simulink model "generate_joint_position_motion"  (R2025a)
settings: Solver=FixedStepDiscrete  StartTime=0.0  StopTime=inf  FixedStep=0.01  RelTol=1e-3
PreLoadFcn:
  | frs = FrankaRobotSettings;
libraries: franka_simulink x1
settings Model: SimulationMode=external  ExtModeTrigDuration=10000  Creator=vasi_ko  LastModifiedBy=kvasios
settings SolverCC: ConcurrentTasks=on  AlgebraicLoopSolver=TrustRegion  AutoInsertRateTranBlk=on
settings DataIOCC: LimitDataPoints=on  SaveFormat=Array  ReturnWorkspaceOutputs=off
settings OptimizationCC: EnhancedBackFolding=on  PassReuseOutputArgsAs=Individual arguments  ZeroExternalMemoryAtStartup=off  ZeroInternalMemoryAtStartup=off  MaxStackSize=200000  OptimizeBlockOrder=speed  DifferentSizesBufferReuse=on  OptimizationCustomize=off  EfficientTunableParamExpr=on
settings DebuggingCC: SolverPrmCheckMsg=warning  ParameterTunabilityLossMsg=error  UnconnectedInputMsg=warning  UnconnectedOutputMsg=warning  UnconnectedLineMsg=warning  SFUnexpectedBacktrackingDiag=warning  SFNoUnconditionalDefaultTransitionDiag=warning  SFExecutionAtInitializationDiag=none  ArithmeticOperatorsInVariantConditions=warning
settings HardwareCC: ProdBitPerLong=64.0  ProdLargestAtomicInteger=LongLong  ProdLargestAtomicFloat=Double  ProdLongLongMode=on  ProdHWDeviceType=ARM Compatible->ARM Cortex-A (64-bit)
settings ModelReferenceCC: EnableRefExpFcnMdlSchedulingChecks=on  PropagateSignalLabelsOutOfModel=off
settings SFSimCC: SimUseLocalCustomCode=off  MATLABDynamicMemAlloc=off  CustomCodeUndefinedFunction=UseInterfaceOnly  SimTargetLang=C++  SimDLTargetLibrary=mkl-dnn
settings RTWCC: SystemTargetFile=ert.tlc  HardwareBoard=NVIDIA Jetson  TLCOptions="-aInlineSetEventsForThisBaseRateFcn=TLC_FALSE -aSuppressMultiTaskScheduler=TLC_FALSE  -aRateBasedStepFcn=0"  TemplateMakefile=ert_default_tmf  RTWVerbose=off  RTWUseLocalCustomCode=off  BuildConfiguration=Faster Runs  TargetLang=C++  GPUComputeCapability=3.5  DLArmComputeVersion=19.05  Description=Embedded Coder
settings CodeAppCC: ForceParamTrailComments=on  IgnoreCustomStorageClasses=off  OperatorAnnotations=on  SimulinkDataObjDesc=on  SFDataObjDesc=on  InsertBlockDesc=on
settings ERTTargetCC: ExtModeTransport=0.0  ExtModeMexFile=ext_comm  ExtModeIntrfLevel=Level1  InlinedParameterPlacement=Hierarchical  RootIOFormat=Structure reference  TargetLangStandard=C++14 (ISO)
settings ConfigComp: CovMetricSettings=dw  CovSaveCumulativeToWorkspaceVar=on  CovSaveSingleToWorkspaceVar=on  CovExternalEMLEnable=off  CovSFcnEnable=off

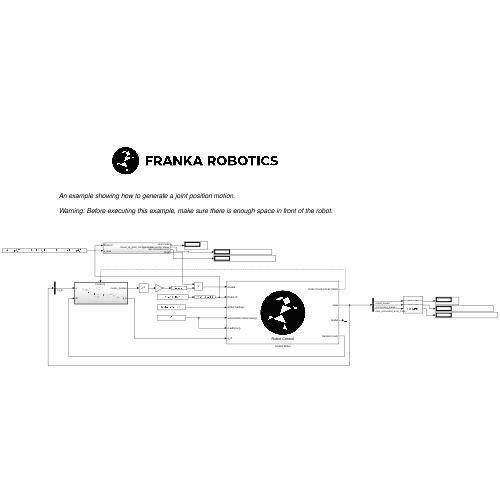
[thumbnail: Simulink's stored preview of the top-level diagram]
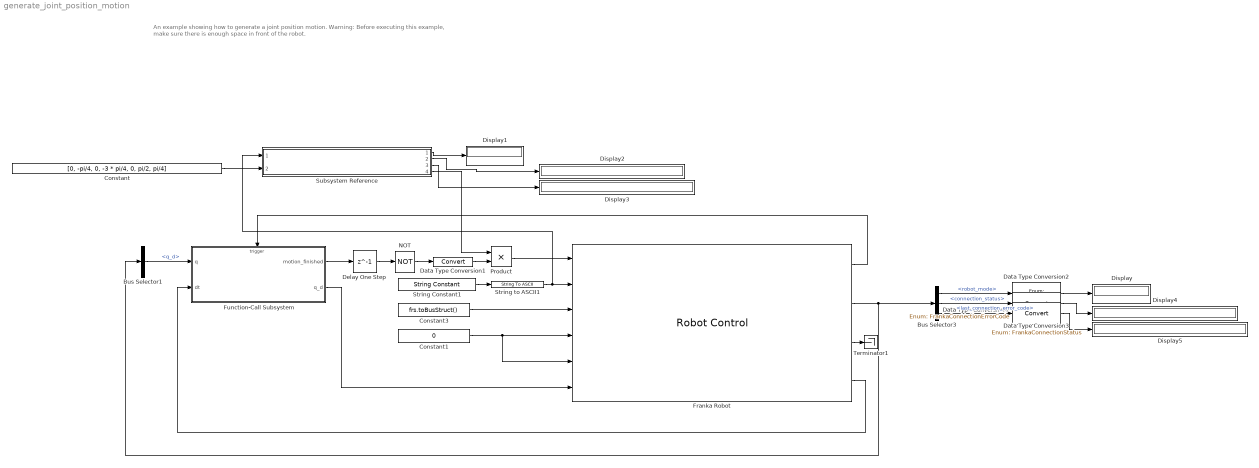
== system generate_joint_position_motion ==
  note: An example showing how to generate a joint position motion.
      |
      | Warning: Before executing this example, make sure there is enough space in front of the robot.
  Bus Selector1 : BusSelector  OutputSignals=q_d
  Bus Selector3 : BusSelector  OutputSignals=robot_mode,connection_status,last_connection_error_code
  Constant : Constant  Value=[0, -pi/4, 0, -3 * pi/4, 0, pi/2, pi/4]
  Constant1 : Constant  Value=0  OutDataTypeStr=Inherit: Inherit via back propagation
  Constant3 : Constant  Value=frs.toBusStruct()  OutDataTypeStr=Bus: FrankaRobotSettingsBus
  Data Type Conversion1 : DataTypeConversion  SaturateOnIntegerOverflow=off  RndMeth=Floor
  Data Type Conversion2 : DataTypeConversion  OutDataTypeStr=Enum: FrankaRobotModes  SaturateOnIntegerOverflow=off  RndMeth=Floor
  Data Type Conversion3 : DataTypeConversion  OutDataTypeStr=Enum: FrankaConnectionStatus  SaturateOnIntegerOverflow=off  RndMeth=Floor
  Data Type Conversion4 : DataTypeConversion  OutDataTypeStr=Enum: FrankaConnectionErrorCode  SaturateOnIntegerOverflow=off  RndMeth=Floor
  Delay One Step : Delay  DelayLength=1
  Display{,1..5} (6 alike) : Display
  Franka Robot : franka_simulink/Robot Control  control_mode=Joint Positions  rt_priority=80  rt_cpu_affinity=-1  rt_lock_memory=off
      settings: SourceProductName=Franka Robotics Simulink Support Package
  Function-Call Subsystem : Subsystem  TreatAsAtomicUnit=on
      settings: RTWSystemCode=Nonreusable function
  NOT : Logic  Operator=NOT  IconShape=distinctive  AllPortsSameDT=off  OutDataTypeStr=boolean
  Product : Product
  String Constant1 : StringConstant  String="\"172.16.0.2\""
  String to ASCII1 : StringToASCII  OutputVectorSize=16
  Subsystem Reference : Subsystem  ReferencedSubsystem=move_to_joint_configuration
  Terminator1 : Terminator
  wires:
  NOT/1 -> Data Type Conversion1/1
  Franka Robot/2 -> Bus Selector3/1, Bus Selector1/1
  Franka Robot/4 -> Function-Call Subsystem/2(dt)
  String to ASCII1/1 -> Subsystem Reference/1, Franka Robot/2
  String Constant1/1 -> String to ASCII1/1
  Function-Call Subsystem/2(q_d) -> Franka Robot/6
  Franka Robot/3 -> Terminator1/1
  Constant3/1 -> Franka Robot/3
  Franka Robot/1 -> Function-Call Subsystem/Trigger
  Bus Selector1/1 -> Function-Call Subsystem/1(q)  "<q_d>"
  Delay One Step/1 -> NOT/1
  Function-Call Subsystem/1(motion_finished) -> Delay One Step/1
  Product/1 -> Franka Robot/1
  Data Type Conversion1/1 -> Product/2
  Constant1/1 -> Franka Robot/5, Franka Robot/4
  Subsystem Reference/1 -> Display1/1
  Constant/1 -> Subsystem Reference/2
  Bus Selector3/2 -> Data Type Conversion3/1  "<connection_status>"
  Data Type Conversion2/1 -> Display/1
  Bus Selector3/1 -> Data Type Conversion2/1  "<robot_mode>"
  Data Type Conversion4/1 -> Display5/1
  Data Type Conversion3/1 -> Display4/1
  Bus Selector3/3 -> Data Type Conversion4/1  "<last_connection_error_code>"
  Subsystem Reference/4 -> Product/1
  Subsystem Reference/2 -> Display2/1
  Subsystem Reference/3 -> Display3/1

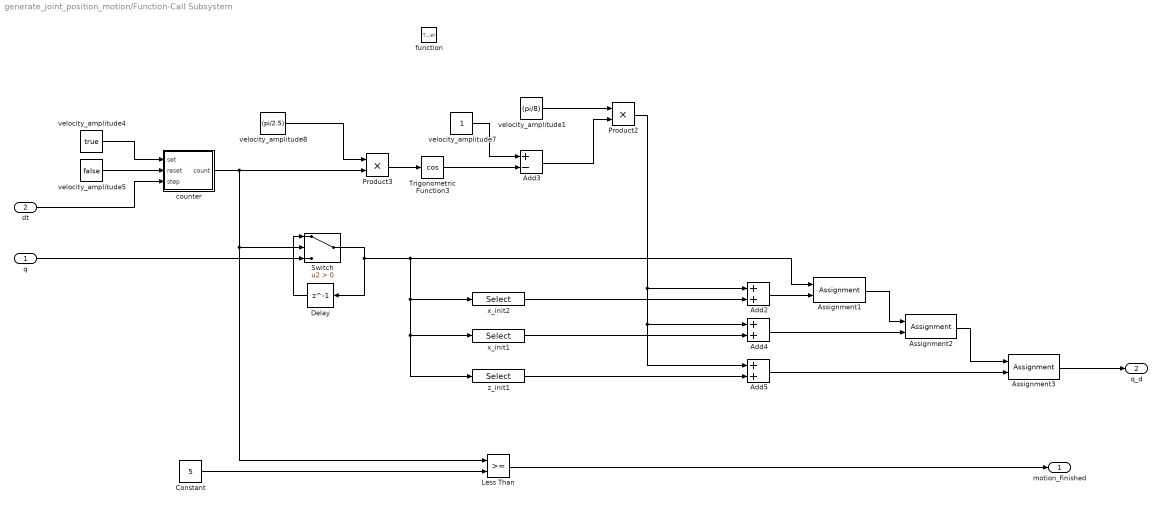
== system generate_joint_position_motion/Function-Call Subsystem ==
  q : Inport
  dt : Inport  Port=2
  function : TriggerPort  TriggerType=function-call  VariantControl=(inherit)
  Add2 : Sum
  Add3 : Sum  Inputs=+-
  Add4 : Sum
  Add5 : Sum
  Assignment1 : Assignment  DiagnosticForDimensions=Warning  IndexOptions=Index vector (dialog)  Indices=4  OutputSizes=1
  Assignment2 : Assignment  DiagnosticForDimensions=Warning  IndexOptions=Index vector (dialog)  Indices=5  OutputSizes=1
  Assignment3 : Assignment  DiagnosticForDimensions=Warning  IndexOptions=Index vector (dialog)  Indices=7  OutputSizes=1
  Constant : Constant  Value=5
  Delay : Delay  DelayLength=1
  Less Than : RelationalOperator  OutDataTypeStr=boolean  RndMeth=Simplest  InputSameDT=off
  Product2 : Product
  Product3 : Product
  Switch : Switch  Criteria=u2 > Threshold  SaturateOnIntegerOverflow=off  InputSameDT=off
  Trigonometric Function3 : Trigonometry  Operator=cos
  counter : Subsystem
  velocity_amplitude1 : Constant  Value=(pi/8)  VectorParams1D=off
  velocity_amplitude4 : Constant  Value=true  VectorParams1D=off
  velocity_amplitude5 : Constant  Value=false  VectorParams1D=off
  velocity_amplitude7 : Constant  VectorParams1D=off
  velocity_amplitude8 : Constant  Value=(pi/2.5)  VectorParams1D=off
  x_init1 : Selector  InputPortWidth=7  IndexOptions=Index vector (dialog)  Indices=5  OutputSizes=1
  x_init2 : Selector  InputPortWidth=7  IndexOptions=Index vector (dialog)  Indices=4  OutputSizes=1
  z_init1 : Selector  InputPortWidth=7  IndexOptions=Index vector (dialog)  Indices=7  OutputSizes=1
  motion_finished : Outport  InitialOutput=0
  q_d : Outport  Port=2  InitialOutput=zeros(7,1)
  wires:
  counter/1(count) -> Product3/2, Switch/2, Less Than/1
  velocity_amplitude5/1 -> counter/2(reset)
  x_init2/1 -> Add2/2
  x_init1/1 -> Add4/2
  q/1 -> Switch/3
  Product2/1 -> Add5/1, Add4/1, Add2/1
  Delay/1 -> Switch/1
  Assignment2/1 -> Assignment3/1
  Product3/1 -> Trigonometric Function3/1
  Add3/1 -> Product2/2
  Assignment1/1 -> Assignment2/1
  velocity_amplitude4/1 -> counter/1(set)
  Add2/1 -> Assignment1/2
  Trigonometric Function3/1 -> Add3/2
  dt/1 -> counter/3(step)
  Assignment3/1 -> q_d/1
  z_init1/1 -> Add5/2
  velocity_amplitude7/1 -> Add3/1
  Switch/1 -> Delay/1, z_init1/1, x_init1/1, x_init2/1, Assignment1/1
  Add5/1 -> Assignment3/2
  Add4/1 -> Assignment2/2
  velocity_amplitude1/1 -> Product2/1
  velocity_amplitude8/1 -> Product3/1
  Constant/1 -> Less Than/2
  Less Than/1 -> motion_finished/1

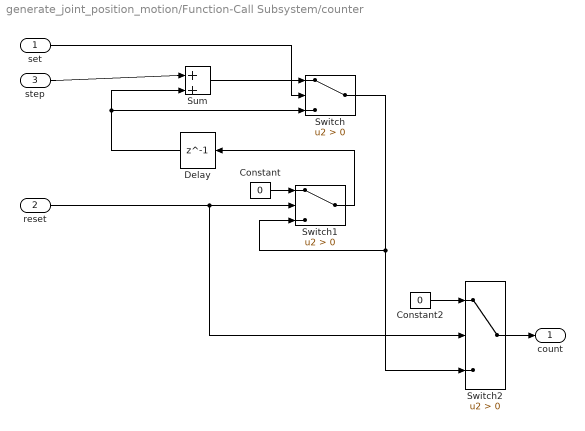
== system generate_joint_position_motion/Function-Call Subsystem/counter ==
  set : Inport  OutDataTypeStr=boolean
  reset : Inport  Port=2  OutDataTypeStr=boolean
  step : Inport  Port=3  OutDataTypeStr=double
  Constant : Constant  Value=0  OutDataTypeStr=double
  Constant2 : Constant  Value=0  OutDataTypeStr=double
  Delay : Delay  DelayLength=1  InitialCondition=0
  Sum : Sum  Inputs=|++
  Switch : Switch  Criteria=u2 > Threshold  SaturateOnIntegerOverflow=off  InputSameDT=off
  Switch1 : Switch  Criteria=u2 > Threshold  OutDataTypeStr=double  SaturateOnIntegerOverflow=off  InputSameDT=off
  Switch2 : Switch  Criteria=u2 > Threshold  OutDataTypeStr=double  SaturateOnIntegerOverflow=off  InputSameDT=off
  count : Outport  OutDataTypeStr=double  VectorParamsAs1DForOutWhenUnconnected=off
  wires:
  Switch2/1 -> count/1
  Constant2/1 -> Switch2/1
  Sum/1 -> Switch/1
  set/1 -> Switch/2
  Switch/1 -> Switch1/3, Switch2/3
  step/1 -> Sum/1
  Delay/1 -> Sum/2, Switch/3
  reset/1 -> Switch1/2, Switch2/2
  Constant/1 -> Switch1/1
  Switch1/1 -> Delay/1
